simulink model "rhszero_discrete_vs_cont_2dof"  (R2014b)
settings: Solver=ode45  StartTime=0.0  StopTime=10  RelTol=1e-3
values from neighbouring files (symbols this model uses):
  aa = exp(-a*h)    [rhszero_variables.m]
  Ffbd = c2d(Ffb, h, 'tustin')    [rhszero_variables.m]
  Fffd = c2d(Fff, h, 'tustin')    [rhszero_variables.m]
  h = 0.05    [BLDC_partial2_fall18.m]    (also in abs_spring18.m = 0.2; active_suspension_ss.m = 0.00416985950901; active_suspension_ss_R.m = 0.00416985950901; active_suspension_ss_spring18.m = 0.004)
  r1 = s0s1r1(3)    [final_dummy.m]
  s0 = 2    [powerplant_dam_controllers.m]
  s1 = -1    [powerplant_dam_controllers.m]
  t0 = subs(Ac, z, 1) / subs(B, z, 1)    [abs_spring18.m]    (also in final_dummy.m = 3.67088607595; harddisk_discrete_design.m = 1/dcgain(Gcb); harddisk_discrete_design_2dof_example.m = 1/dcgain(Gcb))
settings Model: Creator=kjartan  LastModifiedBy=kjartan

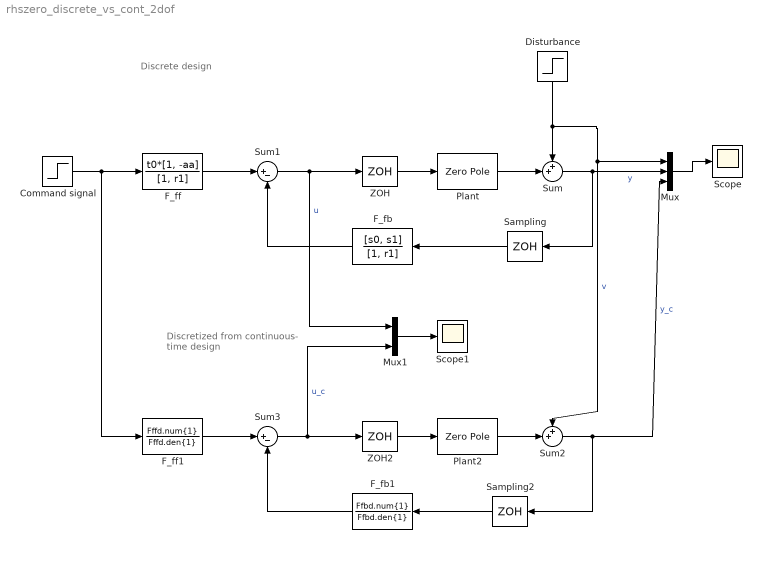
== system rhszero_discrete_vs_cont_2dof ==
  note: Discrete design
  note: Discretized
      | from continuous-
      | time design
  Command signal : Step  Time=0  SampleTime=0
  Disturbance : Step  Time=5  SampleTime=0
  F_fb : DiscreteTransferFcn  Numerator=[s0, s1]  Denominator=[1, r1]  SampleTime=h
  F_fb1 : DiscreteTransferFcn  Numerator=Ffbd.num{1}  Denominator=Ffbd.den{1}  SampleTime=h
  F_ff : DiscreteTransferFcn  Numerator=t0*[1, -aa]  Denominator=[1, r1]  SampleTime=h
  F_ff1 : DiscreteTransferFcn  Numerator=Fffd.num{1}  Denominator=Fffd.den{1}  SampleTime=h
  Mux : Mux  Inputs=3
  Mux1 : Mux  Inputs=2
  Plant : ZeroPole  Zeros=[2]  Poles=[0, -2]  Gain=[-1]
  Plant2 : ZeroPole  Zeros=[2]  Poles=[0, -2]  Gain=[-1]
  Sampling : ZeroOrderHold  SampleTime=h
  Sampling2 : ZeroOrderHold  SampleTime=h
  Scope : Scope
      settings: ShowLegends=on
  Scope1 : Scope
      settings: ShowLegends=on
  Sum : Sum  Inputs=++|
  Sum1 : Sum  Inputs=|+-
  Sum2 : Sum  Inputs=++|
  Sum3 : Sum  Inputs=|+-
  ZOH : ZeroOrderHold  SampleTime=h
  ZOH2 : ZeroOrderHold  SampleTime=h
  wires:
  Sum/1 -> Mux/2, Sampling/1  "y"
  Plant/1 -> Sum/2
  Mux/1 -> Scope/1
  Command signal/1 -> F_ff1/1, F_ff/1
  Disturbance/1 -> Mux/1, Sum2/1, Sum/1  "v"
  Sum1/1 -> Mux1/1, ZOH/1  "u"
  F_fb/1 -> Sum1/2
  F_ff/1 -> Sum1/1
  ZOH/1 -> Plant/1
  Sampling/1 -> F_fb/1
  Sum2/1 -> Mux/3, Sampling2/1  "y_c"
  Plant2/1 -> Sum2/2
  Sum3/1 -> Mux1/2, ZOH2/1  "u_c"
  F_fb1/1 -> Sum3/2
  F_ff1/1 -> Sum3/1
  ZOH2/1 -> Plant2/1
  Sampling2/1 -> F_fb1/1
  Mux1/1 -> Scope1/1
